simulink model "SEIRv4_1"  (R2019b)
settings: Solver=VariableStepAuto  StartTime=0.0  StopTime=365  FixedStep=1/24  RelTol=1e-6
libraries: simulink x2
settings Model: Creator=Alex  LastModifiedBy=Alex

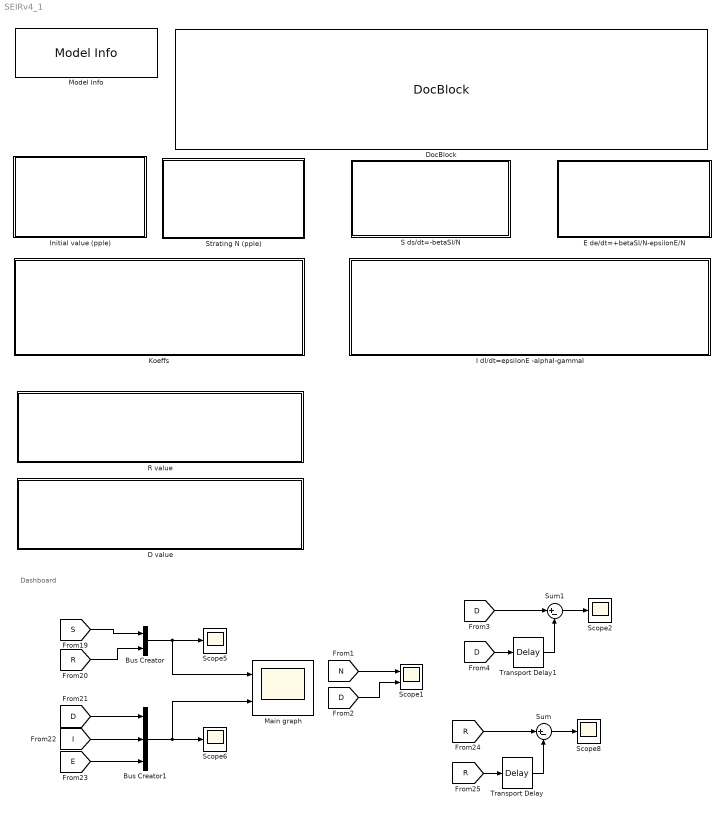
== system SEIRv4_1 ==
  note: Dashboard
  Bus Creator : BusCreator  Inputs=2
  Bus Creator1 : BusCreator  Inputs=3
  D value : Subsystem
  DocBlock : simulink/Model-Wide Utilities/DocBlock  DocumentType=Text
      content=|
      | Классическая SEIR модель с учетом рождаемости и естественной смертности
      |
      | Учитывается смертность, поэтому N (общее количество живого населения в популяции) является переменной во времени.
      |
      | Рождаемость учитывается как lambda N
      | Естественная смертность  как mu S, mu R, mu I (в добавление к смертности от инфекции в SEIRv4), mu R
      |
      | lambda 12.9/1000/365 (данные указаны на 1000 чел за год, а единица моделирования день)
      | mu 12.9/1000/365
      |
      | Для статьи в Резекне 2021
      |
      | На базе этой модели строятся последующие вариации
  E de/dt=+betaSI/N-epsilonE/N : Subsystem
  I dI/dt=epsilonE -alphaI-gammaI : Subsystem
  Initial value (pple) : Subsystem
  Koeffs : Subsystem
  Main graph : Scope  NumInputPorts=2
  Model Info : simulink/Model-Wide Utilities/Model Info  Frame=on  DisplayStringWithTags=|  HorizontalTextAlignment=Left  LeftAlignmentValue=0.02
      | Информация
      | %<Created>
      | %<ModelVersion>
      | %<Description>
  R value : Subsystem
  S ds/dt=-betaSI/N : Subsystem
  Scope1 : Scope  NumInputPorts=2
  Scope{2,5..6,8} (4 alike) : Scope
  Strating N (pple) : Subsystem
  Sum : Sum  Inputs=|+-
  Sum1 : Sum  Inputs=|+-
  Transport Delay : TransportDelay
  Transport Delay1 : TransportDelay
  wires:
  [S] -> Bus Creator/1
  [R] -> Bus Creator/2
  [D] -> Bus Creator1/1
  [I] -> Bus Creator1/2
  [E] -> Bus Creator1/3
  Bus Creator/1 -> Main graph/1, Scope5/1
  Bus Creator1/1 -> Main graph/2, Scope6/1
  [R] -> Transport Delay/1
  [R] -> Sum/1
  Transport Delay/1 -> Sum/2
  Sum/1 -> Scope8/1
  [N] -> Scope1/1
  [D] -> Scope1/2
  Sum1/1 -> Scope2/1
  Transport Delay1/1 -> Sum1/2
  [D] -> Sum1/1
  [D] -> Transport Delay1/1

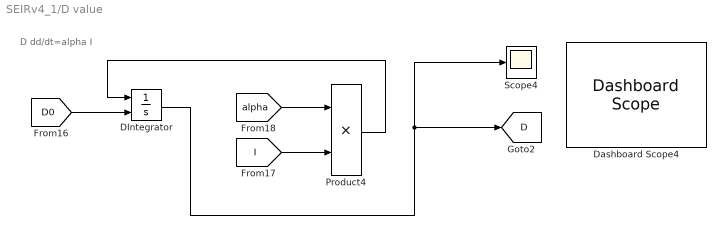
== system SEIRv4_1/D value ==
  note: D dd/dt=alpha I
  DIntegrator : Integrator  InitialConditionSource=external
  Dashboard Scope4 : DashboardScope  Ymax=150e6
  Product4 : Product  Inputs=**
  Scope4 : Scope
  tag scope: D=global
  wires:
  DIntegrator/1 -> [D], Scope4/1
  [I] -> Product4/2
  [alpha] -> Product4/1
  Product4/1 -> DIntegrator/1
  [D0] -> DIntegrator/2

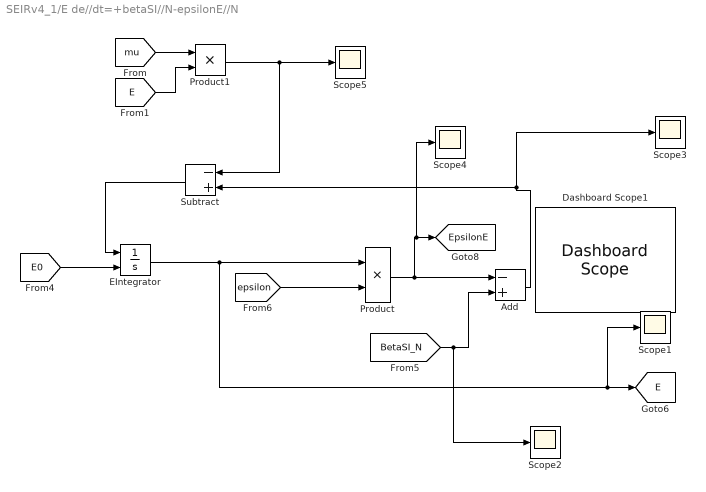
== system SEIRv4_1/E de//dt=+betaSI//N-epsilonE//N ==
  Add : Sum  Inputs=-+
  Dashboard Scope1 : DashboardScope
  EIntegrator : Integrator  InitialConditionSource=external
  Product : Product  Inputs=**
  Product1 : Product
  Scope{1..5} (5 alike) : Scope
  Subtract : Sum  Inputs=-+
  tag scope: E=global, EpsilonE=global
  wires:
  EIntegrator/1 -> Scope1/1, [E], Product/1
  [BetaSI_N] -> Scope2/1, Add/2
  Add/1 -> Subtract/2, Scope3/1
  [epsilon] -> Product/2
  Product/1 -> Scope4/1, [EpsilonE], Add/1
  [E0] -> EIntegrator/2
  [mu] -> Product1/1
  [E] -> Product1/2
  Subtract/1 -> EIntegrator/1
  Product1/1 -> Scope5/1, Subtract/1

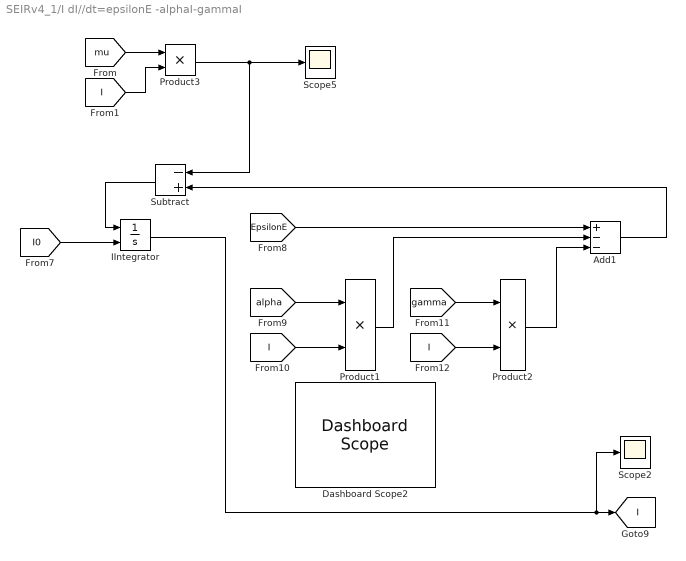
== system SEIRv4_1/I dI//dt=epsilonE -alphaI-gammaI ==
  Add1 : Sum  Inputs=+--
  Dashboard Scope2 : DashboardScope  Ymax=150e6
  IIntegrator : Integrator  InitialConditionSource=external
  Product1 : Product  Inputs=**
  Product2 : Product  Inputs=**
  Product3 : Product
  Scope2 : Scope
  Scope5 : Scope
  Subtract : Sum  Inputs=-+
  tag scope: I=global
  wires:
  [gamma] -> Product2/1
  Product2/1 -> Add1/3
  [EpsilonE] -> Add1/1
  [alpha] -> Product1/1
  Product1/1 -> Add1/2
  IIntegrator/1 -> [I], Scope2/1
  [I] -> Product1/2
  Add1/1 -> Subtract/2
  [I] -> Product2/2
  [I0] -> IIntegrator/2
  [I] -> Product3/2
  Product3/1 -> Scope5/1, Subtract/1
  [mu] -> Product3/1
  Subtract/1 -> IIntegrator/1

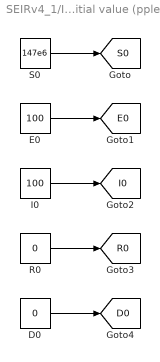
== system SEIRv4_1/Initial value (pple) ==
  D0 : Constant  Value=0
  E0 : Constant  Value=100
  I0 : Constant  Value=100
  R0 : Constant  Value=0
  S0 : Constant  Value=147e6
  tag scope: D0=global, E0=global, I0=global, R0=global, S0=global
  wires:
  S0/1 -> [S0]
  I0/1 -> [I0]
  D0/1 -> [D0]
  E0/1 -> [E0]
  R0/1 -> [R0]

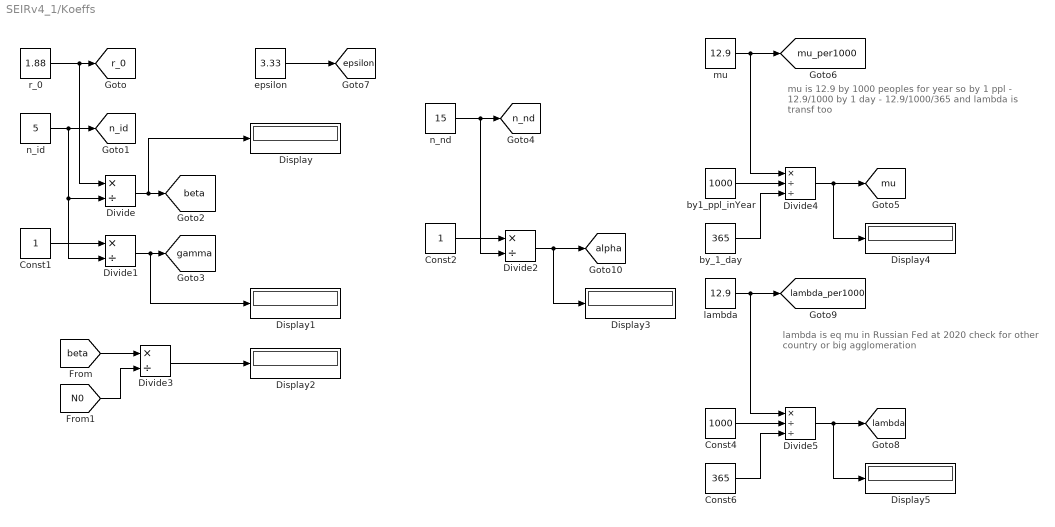
== system SEIRv4_1/Koeffs ==
  note: lambda is eq mu in Russian Fed at 2020
      | check for other country or big agglomeration
  note: mu is 12.9 by 1000 peoples for year
      | so by 1 ppl - 12.9/1000
      | by 1 day - 12.9/1000/365
      | and lambda is transf too
  Const1 : Constant
  Const2 : Constant
  Const4 : Constant  Value=1000
  Const6 : Constant  Value=365
  Display{,1..5} (6 alike) : Display
  Divide{,1..3} (4 alike) : Product  Inputs=*/
  Divide4 : Product  Inputs=*//
  Divide5 : Product  Inputs=*//
  by1_ppl_inYear : Constant  Value=1000
  by_1_day : Constant  Value=365
  epsilon : Constant  Value=3.33
  lambda : Constant  Value=12.9
  mu : Constant  Value=12.9
  n_id : Constant  Value=5
  n_nd : Constant  Value=15
  r_0 : Constant  Value=1.88
  tag scope: alpha=global, beta=global, epsilon=global, gamma=global, lambda=global, lambda_per1000=global, mu=global, mu_per1000=global, n_id=global, n_nd=global, r_0=global
  wires:
  r_0/1 -> Divide/1, [r_0]
  Divide1/1 -> Display1/1, [gamma]
  n_id/1 -> Divide1/2, Divide/2, [n_id]
  Divide/1 -> Display/1, [beta]
  Const1/1 -> Divide1/1
  epsilon/1 -> [epsilon]
  Const2/1 -> Divide2/1
  Divide2/1 -> Display3/1, [alpha]
  n_nd/1 -> [n_nd], Divide2/2
  [beta] -> Divide3/1
  [N0] -> Divide3/2
  Divide3/1 -> Display2/1
  mu/1 -> Divide4/1, [mu_per1000]
  Divide4/1 -> [mu], Display4/1
  by1_ppl_inYear/1 -> Divide4/2
  Const4/1 -> Divide5/2
  Divide5/1 -> Display5/1, [lambda]
  lambda/1 -> [lambda_per1000], Divide5/1
  Const6/1 -> Divide5/3
  by_1_day/1 -> Divide4/3

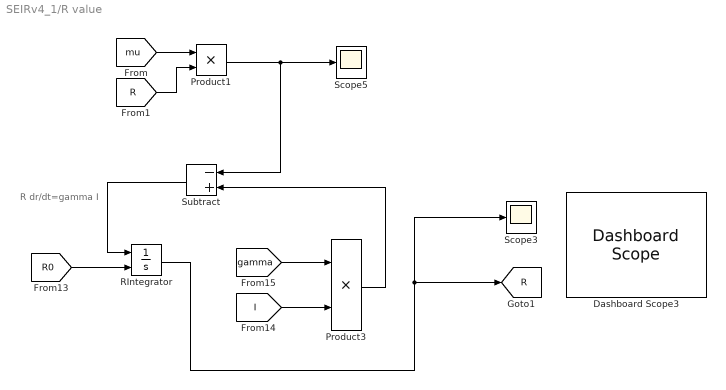
== system SEIRv4_1/R value ==
  note: R dr/dt=gamma I
  Dashboard Scope3 : DashboardScope
  Product1 : Product
  Product3 : Product  Inputs=**
  RIntegrator : Integrator  InitialConditionSource=external
  Scope3 : Scope
  Scope5 : Scope
  Subtract : Sum  Inputs=-+
  tag scope: R=global
  wires:
  Product3/1 -> Subtract/2
  [I] -> Product3/2
  [R0] -> RIntegrator/2
  [gamma] -> Product3/1
  RIntegrator/1 -> Scope3/1, [R]
  [R] -> Product1/2
  Product1/1 -> Scope5/1, Subtract/1
  [mu] -> Product1/1
  Subtract/1 -> RIntegrator/1

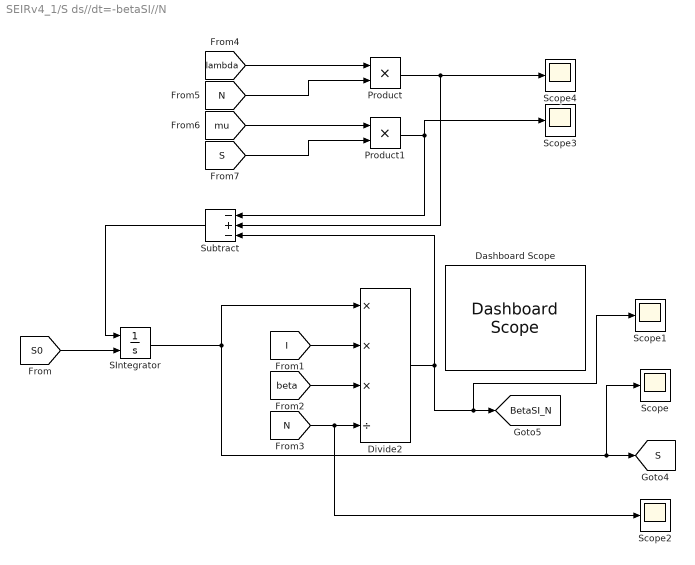
== system SEIRv4_1/S ds//dt=-betaSI//N ==
  Dashboard Scope : DashboardScope  Ymax=150e6
  Divide2 : Product  Inputs=***/
  Product : Product
  Product1 : Product
  SIntegrator : Integrator  InitialConditionSource=external
  Scope{,1..4} (5 alike) : Scope
  Subtract : Sum  Inputs=-+-
  tag scope: BetaSI_N=global, S=global
  wires:
  Divide2/1 -> Subtract/3, Scope1/1, [BetaSI_N]
  SIntegrator/1 -> Scope/1, [S], Divide2/1
  [N] -> Scope2/1, Divide2/4
  [beta] -> Divide2/3
  [I] -> Divide2/2
  [S0] -> SIntegrator/2
  Subtract/1 -> SIntegrator/1
  [mu] -> Product1/1
  [S] -> Product1/2
  Product1/1 -> Subtract/1, Scope3/1
  [lambda] -> Product/1
  [N] -> Product/2
  Product/1 -> Scope4/1, Subtract/2

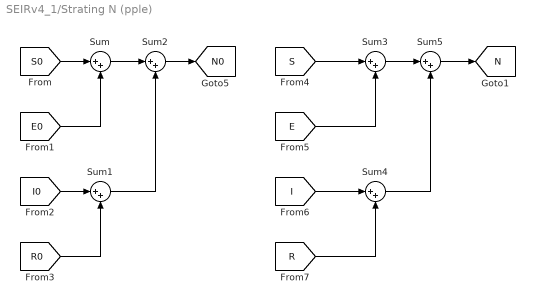
== system SEIRv4_1/Strating N (pple) ==
  Sum{,1..5} (6 alike) : Sum  Inputs=|++
  tag scope: N0=global, N=global
  wires:
  [I0] -> Sum1/1
  [S0] -> Sum/1
  [E0] -> Sum/2
  [R0] -> Sum1/2
  Sum2/1 -> [N0]
  Sum1/1 -> Sum2/2
  Sum/1 -> Sum2/1
  [S] -> Sum3/1
  [E] -> Sum3/2
  [I] -> Sum4/1
  [R] -> Sum4/2
  Sum3/1 -> Sum5/1
  Sum4/1 -> Sum5/2
  Sum5/1 -> [N]
